simulink model "ANC_01"  (R2022a)
settings: Solver=FixedStepDiscrete  StartTime=0.0  StopTime=10  FixedStep=0.001  RelTol=1e-3
undefined symbols (not defined in the file): Filter_Lenth, FS, Sampling_rate
libraries: simulink x3, dspadpt3 x3, dspsrcs4 x2
settings Model: DataDictionary=ModelParameter.sldd  Creator=Administrator  LastModifiedBy=Administrator
settings OptimizationCC: DefaultParameterBehavior=Inlined  EnhancedBackFolding=on  PassReuseOutputArgsAs=Individual arguments  ZeroExternalMemoryAtStartup=off  ZeroInternalMemoryAtStartup=off  OptimizeBlockOrder=speed  DifferentSizesBufferReuse=on  OptimizationCustomize=off  EfficientTunableParamExpr=on
settings DebuggingCC: ParameterTunabilityLossMsg=error
settings SFSimCC: MATLABDynamicMemAlloc=off
settings RTWCC: SystemTargetFile=ert.tlc  TemplateMakefile=ert_default_tmf  GenerateReport=on  LaunchReport=on
settings CodeAppCC: ForceParamTrailComments=on  IgnoreCustomStorageClasses=off  OperatorAnnotations=on  SimulinkDataObjDesc=on  SFDataObjDesc=on  InsertBlockDesc=on
settings ERTTargetCC: TargetLangStandard=C99 (ISO)  GenerateSampleERTMain=on  InlinedParameterPlacement=NonHierarchical  ERTCustomFileTemplate=example_file_process.tlc

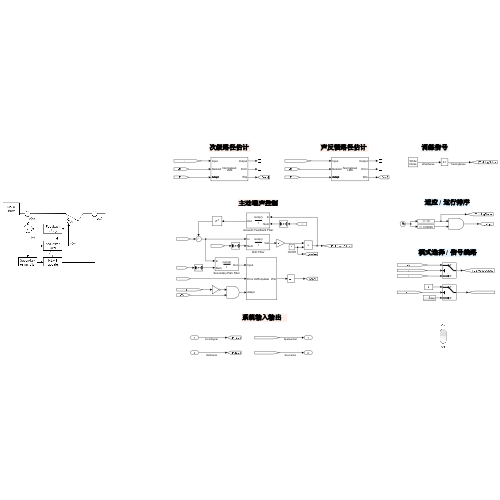
[thumbnail: Simulink's stored preview of the top-level diagram]
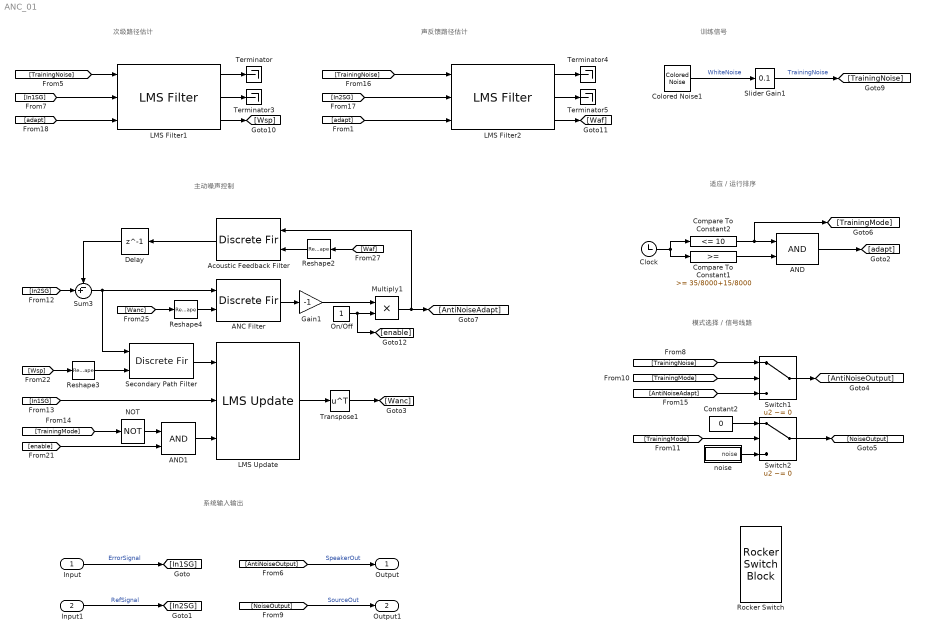
== system ANC_01 ==
  note: 声反馈路径估计
  note: 次级路径估计
  note: 主动噪声控制
  note: 模式选择 / 信号线路
  note: 训练信号
  note: 适应 / 运行排序
  note: 系统输入输出
  Input : Inport
  Input1 : Inport  Port=2
  ANC Filter : DiscreteFir  CoefSource=Input port
      settings: InputPortMap=u0,u1
  AND : Logic  IconShape=distinctive  AllPortsSameDT=off  OutDataTypeStr=boolean
  AND1 : Logic  IconShape=distinctive  AllPortsSameDT=off  OutDataTypeStr=boolean
  Acoustic Feedback Filter : DiscreteFir  CoefSource=Input port
      settings: InputPortMap=u0,u1
  Clock : Clock
  Colored Noise1 : dspsrcs4/Colored Noise  Color=white  InverseFrequencyPower=0.5  BoundedOutput=off  NumChannels=1  OutputDataType=double  SamplesPerFrame=1  SampleTime=1/Sampling_rate  RandomStream=mt19937ar with seed  Seed=67  SimulateUsing=Code generation
      settings: SourceProductBaseCode=DS
  Compare To Constant1 : simulink/Logic and Bit Operations/Compare To Constant  relop=>=  const=35/8000+15/8000  OutDataTypeStr=boolean
  Compare To Constant2 : simulink/Logic and Bit Operations/Compare To Constant  relop=<=  const=10  OutDataTypeStr=boolean
  Constant2 : Constant  Value=0
  Delay : Delay  DelayLength=1
  Gain1 : Gain  Gain=-1
  LMS Filter1 : dspadpt3/LMS Filter  Algo=Normalized LMS  L=Filter_Lenth/2  stepflag=Dialog  mu=0.02  leakage=1.0  ic=0  Adapt=on  resetflag=None  weights=on  addnparflag=off  roundingMode=Floor  overflowMode=off
      settings: SourceProductBaseCode=DS
  LMS Filter2 : dspadpt3/LMS Filter  Algo=Normalized LMS  L=Filter_Lenth/2  stepflag=Dialog  mu=0.02  leakage=1.0  ic=0  Adapt=on  resetflag=None  weights=on  addnparflag=off  roundingMode=Floor  overflowMode=off
      settings: SourceProductBaseCode=DS
  LMS Update : dspadpt3/LMS Update  Method=Normalized LMS  Length=Filter_Lenth  NumFilters=1  StepSizeSource=Property  StepSize=0.002  LeakageFactor=1.0  InitialConditions=0  AdaptiveFilterMode=Tapped delay-line FIR filter  EnableAdaptInput=on  EnableResetInput=off  SimulateUsing=Code generation
      settings: SourceProductBaseCode=DS
  Multiply1 : Product
  NOT : Logic  Operator=NOT  IconShape=distinctive  AllPortsSameDT=off  OutDataTypeStr=boolean
  On/Off : Constant
  Reshape2 : Reshape  OutputDimensionality=Row vector (2-D)
  Reshape3 : Reshape  OutputDimensionality=Row vector (2-D)
  Reshape4 : Reshape  OutputDimensionality=Row vector (2-D)
  Rocker Switch : RockerSwitchBlock  LabelPosition=Hide
      settings: Values={{'Off', 'On'}, [0 1]}
  Secondary Path Filter : DiscreteFir  CoefSource=Input port
      settings: InputPortMap=u0,u1
  Slider Gain1 : simulink/Math Operations/Slider Gain  gain=0.1  low=0  high=1
  Sum3 : Sum  Inputs=-+|
  Switch1 : Switch  Criteria=u2 ~= 0  Threshold=5  SaturateOnIntegerOverflow=off  InputSameDT=off
  Switch2 : Switch  Criteria=u2 ~= 0  Threshold=5  SaturateOnIntegerOverflow=off  InputSameDT=off
  Terminator{,3..5} (4 alike) : Terminator
  Transpose1 : Math  Operator=transpose  SignedPower=on
  noise : Subsystem
  Output : Outport
  Output1 : Outport  Port=2
  wires:
  Colored Noise1/1 -> Slider Gain1/1  "WhiteNoise"
  [enable] -> AND1/2
  noise/1(noise) -> Switch2/3
  [adapt] -> LMS Filter1/3
  Clock/1 -> Compare To Constant2/1, Compare To Constant1/1
  Gain1/1 -> Multiply1/1
  LMS Update/1 -> Transpose1/1
  Acoustic Feedback Filter/1 -> Delay/1
  Switch1/1 -> [AntiNoiseOutput]
  Constant2/1 -> Switch2/1
  [AntiNoiseAdapt] -> Switch1/3
  LMS Filter1/2 -> Terminator3/1
  LMS Filter2/3 -> [Waf]
  LMS Filter2/2 -> Terminator5/1
  [adapt] -> LMS Filter2/3
  [In1SG] -> LMS Filter1/2
  LMS Filter1/3 -> [Wsp]
  [In2SG] -> Sum3/2
  [TrainingMode] -> Switch1/2
  LMS Filter2/1 -> Terminator4/1
  Compare To Constant1/1 -> AND/2
  Secondary Path Filter/1 -> LMS Update/1
  On/Off/1 -> Multiply1/2, [enable]
  [TrainingNoise] -> LMS Filter1/1
  Compare To Constant2/1 -> [TrainingMode], AND/1
  [TrainingMode] -> NOT/1
  AND1/1 -> LMS Update/3
  Transpose1/1 -> [Wanc]
  Slider Gain1/1 -> [TrainingNoise]  "TrainingNoise"
  Multiply1/1 -> Acoustic Feedback Filter/1, [AntiNoiseAdapt]
  Input1/1 -> [In2SG]  "RefSignal"
  NOT/1 -> AND1/1
  [TrainingNoise] -> Switch1/1
  [In2SG] -> LMS Filter2/2
  LMS Filter1/1 -> Terminator/1
  Switch2/1 -> [NoiseOutput]
  [In1SG] -> LMS Update/2
  Input/1 -> [In1SG]  "ErrorSignal"
  ANC Filter/1 -> Gain1/1
  [TrainingMode] -> Switch2/2
  AND/1 -> [adapt]
  [AntiNoiseOutput] -> Output/1  "SpeakerOut"
  [NoiseOutput] -> Output1/1  "SourceOut"
  [TrainingNoise] -> LMS Filter2/1
  [Waf] -> Reshape2/1
  Reshape2/1 -> Acoustic Feedback Filter/2
  Sum3/1 -> Secondary Path Filter/1, ANC Filter/1
  [Wsp] -> Reshape3/1
  Reshape3/1 -> Secondary Path Filter/2
  [Wanc] -> Reshape4/1
  Reshape4/1 -> ANC Filter/2
  Delay/1 -> Sum3/1

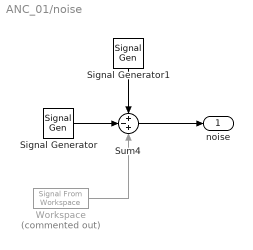
== system ANC_01/noise ==
  Signal Generator : SignalGenerator  Amplitude=.2  Frequency=150
  Signal Generator1 : SignalGenerator  Amplitude=.15  Frequency=225
  Sum4 : Sum  Inputs=+-+
  Workspace : dspsrcs4/Signal From Workspace  Commented=on  X=noise  Ts=1/FS  nsamps=1  OutputAfterFinalValue=Cyclic repetition  ignoreOrWarnInputAndFrameLengths=off  OutputFrames=off
  noise : Outport  VectorParamsAs1DForOutWhenUnconnected=off
  wires:
  Signal Generator/1 -> Sum4/2
  Signal Generator1/1 -> Sum4/1
  Sum4/1 -> noise/1
  Workspace/1 -> Sum4/3
